simulink model "displayAlgorithm"  (R2015a)
settings: Solver=ode45  StartTime=0.0  StopTime=inf  RelTol=1e-3
InitFcn:
  | load busObjects
undefined symbols (not defined in the file or in its folder): gray
libraries: visiontextngfix x10, visionsinks x2, dspvision x1, sldrtlib x1
settings Model: Creator=sbiagion  LastModifiedBy=sbiagion
settings DebuggingCC: UnderspecifiedInitializationDetection=Classic  MergeDetectMultiDrivingBlocksExec=none  SolverPrmCheckMsg=warning

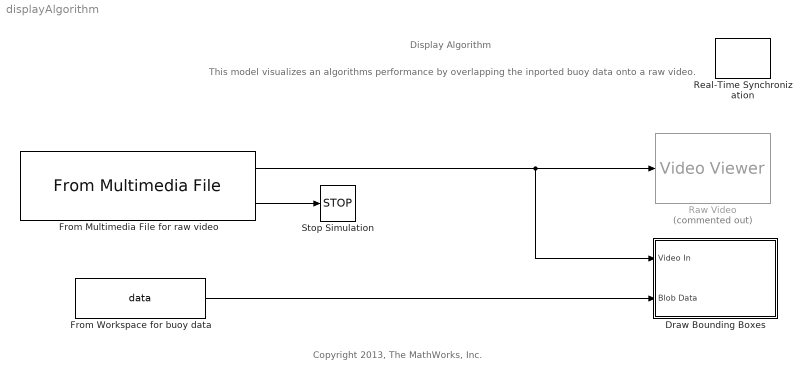
== system displayAlgorithm ==
  note: Copyright 2013, The MathWorks, Inc.
  note: This model visualizes an algorithms performance by overlapping the inported buoy data onto a raw video.
  note: Display Algorithm
  Draw Bounding Boxes : Subsystem
  From Multimedia File for raw video : dspvision/From Multimedia File  inputFilename=..\media\rawVideo_640x480.avi  loop=on  numPlays=1  outputStreams=Video only  videoDataType=uint8  audioDataType=int16  inheritSampleTime=on  userDefinedSampleTime=0.1  noAudioOutput=off  isIntensityVideo=off  fourcc=RGB  colorVideoFormat=One multidimensional signal  outputEOF=on  dataOrg=Column-major  audioFrameSize=1024  computeAudioFrameSize=off  outSamplingMode=Sample based
  From Workspace for buoy data : FromWorkspace  VariableName=data  OutDataTypeStr=Bus: dataBusObject
  "Raw Video " : visionsinks/Video Viewer  Commented=on  inputType=Obsolete7b  imagePorts=One multidimensional signal  useColorMap=off  colormapValue=gray(256)  specRange=off  minInputVal=0  maxInputVal=255  FigPos=[880 975 1008 708]  AxisZoom=on  trueSizedOnce=off  OpenAtMdlStart=on  DefaultConfigurationName=vipscopes.VideoViewerScopeCfg
  Real-Time Synchronization : sldrtlib/Real-Time Synchronization  SampleTime=0.1  MaxMissedTicks=1e9  ShowMissedTicks=off  YieldWhenWaiting=off
  Stop Simulation : Stop
  wires:
  From Workspace for buoy data/1 -> Draw Bounding Boxes/2(Blob Data)
  From Multimedia File for raw video/1 -> Draw Bounding Boxes/1(Video In), "Raw Video "/1
  From Multimedia File for raw video/2 -> Stop Simulation/1

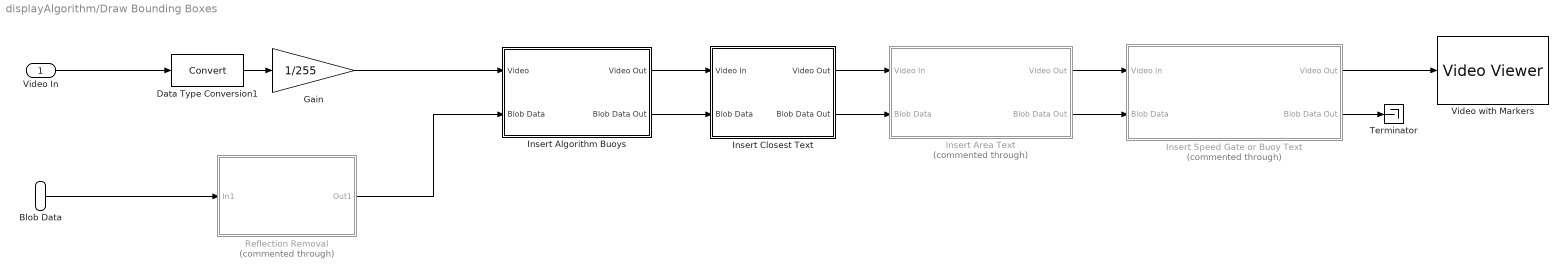
== system displayAlgorithm/Draw Bounding Boxes ==
  Video In : Inport
  Blob Data : Inport  Port=2
  Data Type Conversion1 : DataTypeConversion
  Gain : Gain  Gain=1/255
  Insert Algorithm Buoys : Subsystem
  Insert Area Text : Subsystem  Commented=through
  Insert Closest Text : Subsystem
  Insert Speed Gate or Buoy Text : Subsystem  Commented=through
  Reflection Removal : Subsystem  Commented=through
  Terminator : Terminator
  Video with Markers : visionsinks/Video Viewer  inputType=Obsolete7b  imagePorts=One multidimensional signal  useColorMap=off  colormapValue=gray(256)  specRange=off  minInputVal=0  maxInputVal=255  FigPos=[7 972 845 656]  AxisZoom=on  trueSizedOnce=off  OpenAtMdlStart=on  DefaultConfigurationName=vipscopes.VideoViewerScopeCfg
  wires:
  Data Type Conversion1/1 -> Gain/1
  Video In/1 -> Data Type Conversion1/1
  Insert Speed Gate or Buoy Text/1(Video Out) -> Video with Markers/1
  Insert Area Text/1(Video Out) -> Insert Speed Gate or Buoy Text/1(Video In)
  Insert Closest Text/1(Video Out) -> Insert Area Text/1(Video In)
  Reflection Removal/1(Out1) -> Insert Algorithm Buoys/2(Blob Data)
  Blob Data/1 -> Reflection Removal/1(In1)
  Gain/1 -> Insert Algorithm Buoys/1(Video)
  Insert Algorithm Buoys/1(Video Out) -> Insert Closest Text/1(Video In)
  Insert Algorithm Buoys/2(Blob Data Out) -> Insert Closest Text/2(Blob Data)
  Insert Closest Text/2(Blob Data Out) -> Insert Area Text/2(Blob Data)
  Insert Area Text/2(Blob Data Out) -> Insert Speed Gate or Buoy Text/2(Blob Data)
  Insert Speed Gate or Buoy Text/2(Blob Data Out) -> Terminator/1

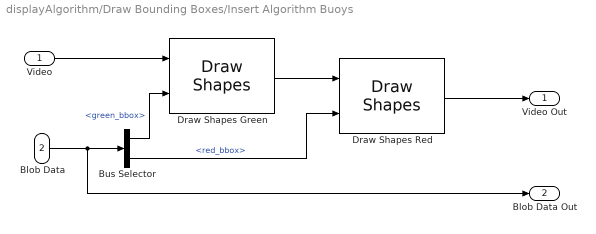
== system displayAlgorithm/Draw Bounding Boxes/Insert Algorithm Buoys ==
  Video : Inport
  Blob Data : Inport  Port=2
  Bus Selector : BusSelector  OutputSignals=green_bbox,red_bbox
  Draw Shapes Green : visiontextngfix/Draw Shapes  shape=Rectangles  fill=on  fillClrSource=Specify via dialog  display=User-specified value  intensity=200  color=[0 255 0]  opacity=0.6  viewport=Entire image  antialiasing=off  inType=Obsolete  imagePorts=One multidimensional signal  prodOutputMode=Binary point scaling  prodOutputWordLength=32  prodOutputFracLength=14  memoryMode=Specify word length  memoryWordLength=16  memoryFracLength=14  roundingMode=Floor  overflowMode=off
  Draw Shapes Red : visiontextngfix/Draw Shapes  shape=Rectangles  fill=on  fillClrSource=Specify via dialog  display=User-specified value  intensity=200  color=[255 0 0]  opacity=0.6  viewport=Entire image  antialiasing=off  inType=Obsolete  imagePorts=One multidimensional signal  prodOutputMode=Binary point scaling  prodOutputWordLength=32  prodOutputFracLength=14  memoryMode=Specify word length  memoryWordLength=16  memoryFracLength=14  roundingMode=Floor  overflowMode=off
  Video Out : Outport
  Blob Data Out : Outport  Port=2
  wires:
  Blob Data/1 -> Blob Data Out/1, Bus Selector/1
  Video/1 -> Draw Shapes Green/1
  Draw Shapes Green/1 -> Draw Shapes Red/1
  Draw Shapes Red/1 -> Video Out/1
  Bus Selector/1 -> Draw Shapes Green/2  "<green_bbox>"
  Bus Selector/2 -> Draw Shapes Red/2  "<red_bbox>"

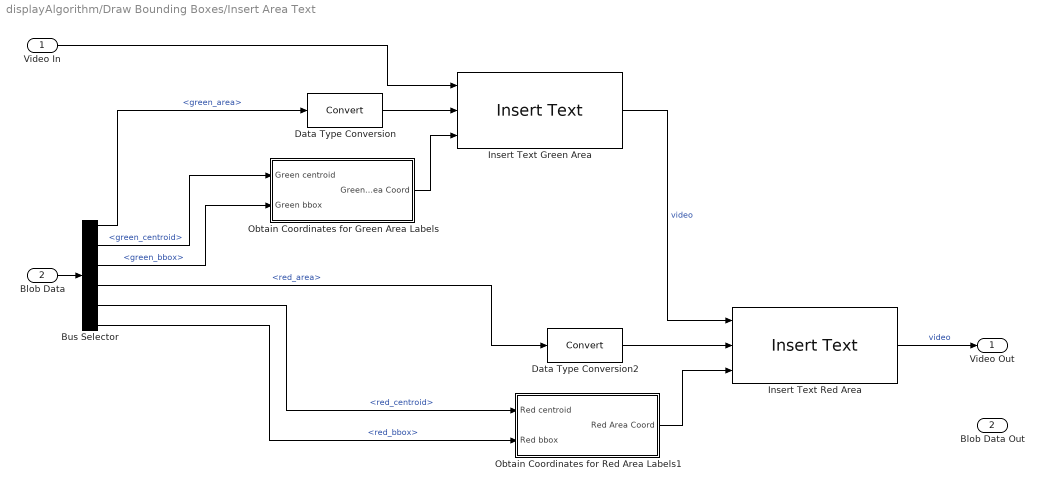
== system displayAlgorithm/Draw Bounding Boxes/Insert Area Text ==
  Video In : Inport
  Blob Data : Inport  Port=2
  Bus Selector : BusSelector  OutputSignals=green_area,green_centroid,green_bbox,red_area,red_centroid,red_bbox
  Data Type Conversion : DataTypeConversion
  Data Type Conversion2 : DataTypeConversion
  Insert Text Green Area : visiontextngfix/Insert Text  inputType=Obsolete  theText='Area: %d'  fontFace=LucidaSansRegular  dummyVar1=0  blockFontSize=12  antiAliased=on  getTextLocFrom=Input port  textLoc=[1 1]  getTextColorFrom=Specify via dialog  textColor=[0 255 0]  getTextIntensityFrom=Specify via dialog  textIntensity=0  getTextOpacityFrom=Specify via dialog  textOpacity=1.0  dummyVar2=0  dummyVar3=0  dummyVar4=0  imagePorts=One multidimensional signal  isInputTransposed=off
  Insert Text Red Area : visiontextngfix/Insert Text  inputType=Obsolete  theText='Area: %d'  fontFace=LucidaSansRegular  dummyVar1=0  blockFontSize=12  antiAliased=on  getTextLocFrom=Input port  textLoc=[1 1]  getTextColorFrom=Specify via dialog  textColor=[255 0 0]  getTextIntensityFrom=Specify via dialog  textIntensity=0  getTextOpacityFrom=Specify via dialog  textOpacity=1.0  dummyVar2=0  dummyVar3=0  dummyVar4=0  imagePorts=One multidimensional signal  isInputTransposed=off
  Obtain Coordinates for Green Area Labels : Subsystem
  Obtain Coordinates for Red Area Labels1 : Subsystem
  Video Out : Outport
  Blob Data Out : Outport  Port=2
  wires:
  Insert Text Red Area/1 -> Video Out/1  "video"
  Video In/1 -> Insert Text Green Area/1
  Bus Selector/4 -> Data Type Conversion2/1  "<red_area>"
  Bus Selector/1 -> Data Type Conversion/1  "<green_area>"
  Data Type Conversion/1 -> Insert Text Green Area/2
  Obtain Coordinates for Red Area Labels1/1(Red Area Coord) -> Insert Text Red Area/3
  Insert Text Green Area/1 -> Insert Text Red Area/1  "video"
  Data Type Conversion2/1 -> Insert Text Red Area/2
  Obtain Coordinates for Green Area Labels/1(Green Area Coord) -> Insert Text Green Area/3
  Blob Data/1 -> Bus Selector/1
  Bus Selector/2 -> Obtain Coordinates for Green Area Labels/1(Green centroid)  "<green_centroid>"
  Bus Selector/3 -> Obtain Coordinates for Green Area Labels/2(Green bbox)  "<green_bbox>"
  Bus Selector/5 -> Obtain Coordinates for Red Area Labels1/1(Red centroid)  "<red_centroid>"
  Bus Selector/6 -> Obtain Coordinates for Red Area Labels1/2(Red bbox)  "<red_bbox>"

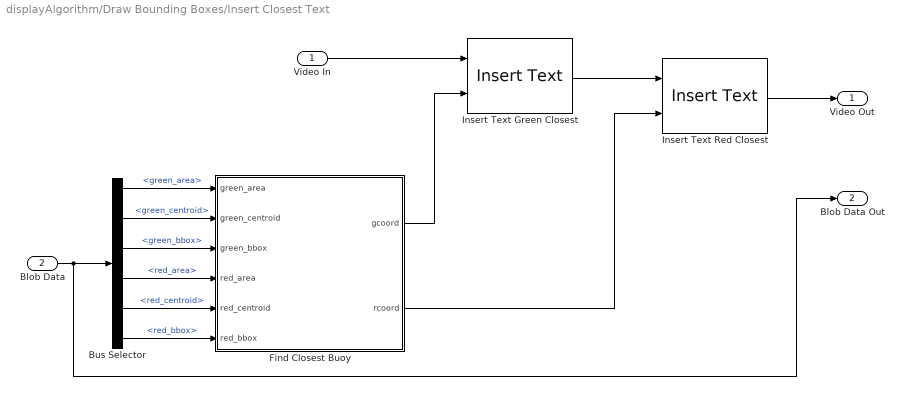
== system displayAlgorithm/Draw Bounding Boxes/Insert Closest Text ==
  Video In : Inport
  Blob Data : Inport  Port=2
  Bus Selector : BusSelector  OutputSignals=green_area,green_centroid,green_bbox,red_area,red_centroid,red_bbox
  Find Closest Buoy : MATLAB Function  TreatAsAtomicUnit=on
  Insert Text Green Closest : visiontextngfix/Insert Text  inputType=Obsolete  theText='Closest Green Buoy'  fontFace=LucidaSansRegular  dummyVar1=0  blockFontSize=12  antiAliased=on  getTextLocFrom=Input port  textLoc=[1 1]  getTextColorFrom=Specify via dialog  textColor=[0 255 0]  getTextIntensityFrom=Specify via dialog  textIntensity=0  getTextOpacityFrom=Specify via dialog  textOpacity=1.0  dummyVar2=0  dummyVar3=0  dummyVar4=0  imagePorts=One multidimensional signal  isInputTransposed=off
  Insert Text Red Closest : visiontextngfix/Insert Text  inputType=Obsolete  theText='Closest Red Buoy'  fontFace=LucidaSansRegular  dummyVar1=0  blockFontSize=12  antiAliased=on  getTextLocFrom=Input port  textLoc=[1 1]  getTextColorFrom=Specify via dialog  textColor=[255 0 0]  getTextIntensityFrom=Specify via dialog  textIntensity=0  getTextOpacityFrom=Specify via dialog  textOpacity=1.0  dummyVar2=0  dummyVar3=0  dummyVar4=0  imagePorts=One multidimensional signal  isInputTransposed=off
  Video Out : Outport
  Blob Data Out : Outport  Port=2
  wires:
  Insert Text Green Closest/1 -> Insert Text Red Closest/1
  Video In/1 -> Insert Text Green Closest/1
  Insert Text Red Closest/1 -> Video Out/1
  Find Closest Buoy/1(gcoord) -> Insert Text Green Closest/2
  Find Closest Buoy/2(rcoord) -> Insert Text Red Closest/2
  Blob Data/1 -> Blob Data Out/1, Bus Selector/1
  Bus Selector/3 -> Find Closest Buoy/3(green_bbox)  "<green_bbox>"
  Bus Selector/4 -> Find Closest Buoy/4(red_area)  "<red_area>"
  Bus Selector/2 -> Find Closest Buoy/2(green_centroid)  "<green_centroid>"
  Bus Selector/5 -> Find Closest Buoy/5(red_centroid)  "<red_centroid>"
  Bus Selector/1 -> Find Closest Buoy/1(green_area)  "<green_area>"
  Bus Selector/6 -> Find Closest Buoy/6(red_bbox)  "<red_bbox>"

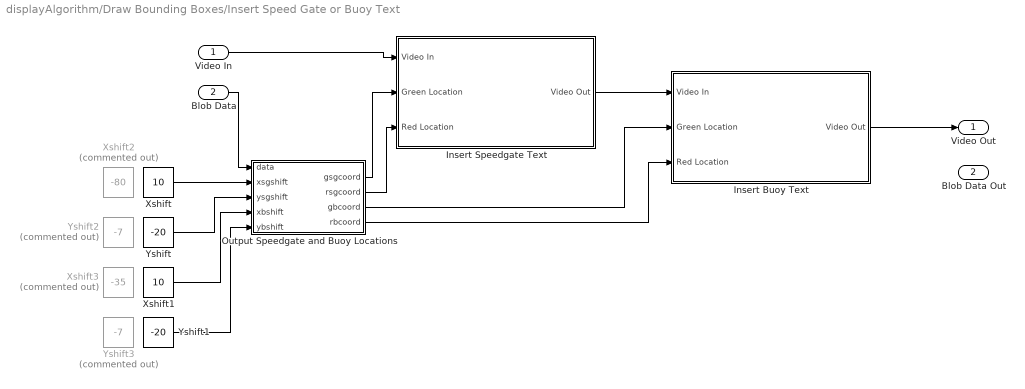
== system displayAlgorithm/Draw Bounding Boxes/Insert Speed Gate or Buoy Text ==
  Video In : Inport
  Blob Data : Inport  Port=2
  Insert Buoy Text : Subsystem
  Insert Speedgate Text : Subsystem
  Output Speedgate and Buoy Locations : MATLAB Function  TreatAsAtomicUnit=on
  Xshift : Constant  Value=10
  Xshift1 : Constant  Value=10
  Xshift2 : Constant  Commented=on  Value=-80
  Xshift3 : Constant  Commented=on  Value=-35
  Yshift : Constant  Value=-20
  Yshift1 : Constant  Value=-20
  Yshift2 : Constant  Commented=on  Value=-7
  Yshift3 : Constant  Commented=on  Value=-7
  Video Out : Outport
  Blob Data Out : Outport  Port=2
  wires:
  Video In/1 -> Insert Speedgate Text/1(Video In)
  Insert Speedgate Text/1(Video Out) -> Insert Buoy Text/1(Video In)
  Insert Buoy Text/1(Video Out) -> Video Out/1
  Blob Data/1 -> Output Speedgate and Buoy Locations/1(data)
  Output Speedgate and Buoy Locations/1(gsgcoord) -> Insert Speedgate Text/2(Green Location)
  Output Speedgate and Buoy Locations/2(rsgcoord) -> Insert Speedgate Text/3(Red Location)
  Output Speedgate and Buoy Locations/3(gbcoord) -> Insert Buoy Text/2(Green Location)
  Output Speedgate and Buoy Locations/4(rbcoord) -> Insert Buoy Text/3(Red Location)
  Xshift/1 -> Output Speedgate and Buoy Locations/2(xsgshift)
  Yshift/1 -> Output Speedgate and Buoy Locations/3(ysgshift)
  Xshift1/1 -> Output Speedgate and Buoy Locations/4(xbshift)
  Yshift1/1 -> Output Speedgate and Buoy Locations/5(ybshift)

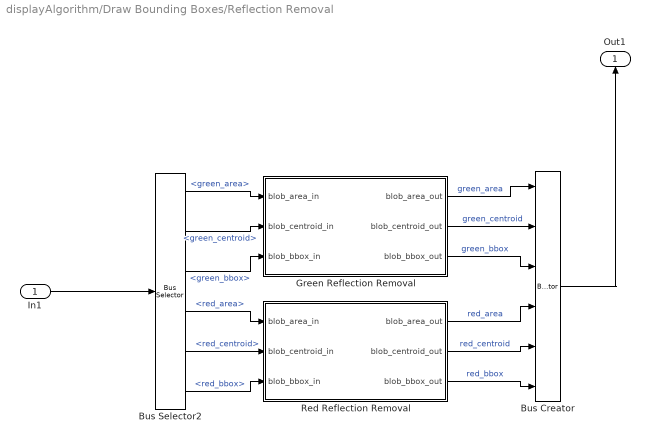
== system displayAlgorithm/Draw Bounding Boxes/Reflection Removal ==
  In1 : Inport
  Bus Creator : BusCreator  Inputs=6
  Bus Selector2 : BusSelector  OutputSignals=green_area,green_centroid,green_bbox,red_area,red_centroid,red_bbox
  Green Reflection Removal : MATLAB Function  TreatAsAtomicUnit=on
  Red Reflection Removal : MATLAB Function  TreatAsAtomicUnit=on
  Out1 : Outport
  wires:
  Red Reflection Removal/3(blob_bbox_out) -> Bus Creator/6  "red_bbox"
  Bus Selector2/1 -> Green Reflection Removal/1(blob_area_in)  "<green_area>"
  In1/1 -> Bus Selector2/1
  Bus Selector2/2 -> Green Reflection Removal/2(blob_centroid_in)  "<green_centroid>"
  Bus Selector2/4 -> Red Reflection Removal/1(blob_area_in)  "<red_area>"
  Bus Selector2/6 -> Red Reflection Removal/3(blob_bbox_in)  "<red_bbox>"
  Red Reflection Removal/2(blob_centroid_out) -> Bus Creator/5  "red_centroid"
  Green Reflection Removal/3(blob_bbox_out) -> Bus Creator/3  "green_bbox"
  Red Reflection Removal/1(blob_area_out) -> Bus Creator/4  "red_area"
  Bus Selector2/5 -> Red Reflection Removal/2(blob_centroid_in)  "<red_centroid>"
  Bus Creator/1 -> Out1/1
  Green Reflection Removal/1(blob_area_out) -> Bus Creator/1  "green_area"
  Bus Selector2/3 -> Green Reflection Removal/3(blob_bbox_in)  "<green_bbox>"
  Green Reflection Removal/2(blob_centroid_out) -> Bus Creator/2  "green_centroid"

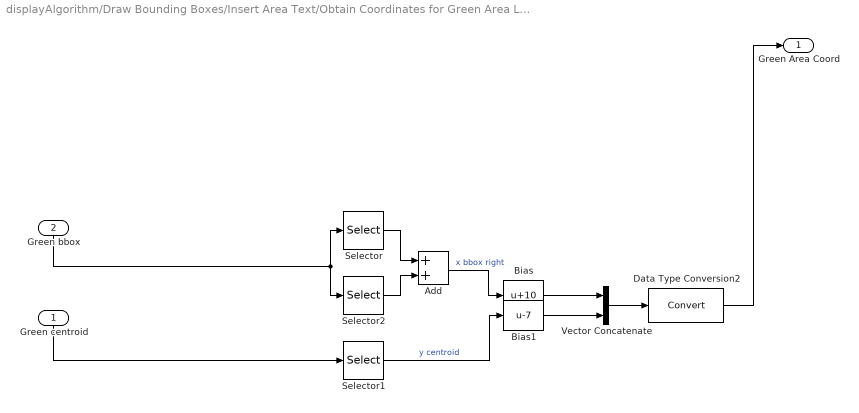
== system displayAlgorithm/Draw Bounding Boxes/Insert Area Text/Obtain Coordinates for Green Area Labels ==
  Green centroid : Inport
  Green bbox : Inport  Port=2
  Add : Sum
  Bias : Bias  Bias=10
  Bias1 : Bias  Bias=-7
  Data Type Conversion2 : DataTypeConversion
  Selector : Selector  NumberOfDimensions=2  InputPortWidth=3  IndexOptions=Select all,Index vector (dialog)  Indices=[1 3],1  OutputSizes=1,1
  Selector1 : Selector  NumberOfDimensions=2  InputPortWidth=3  IndexOptions=Select all,Index vector (dialog)  Indices=[1 3],2  OutputSizes=1,1
  Selector2 : Selector  NumberOfDimensions=2  InputPortWidth=3  IndexOptions=Select all,Index vector (dialog)  Indices=[1 3],3  OutputSizes=1,1
  Vector Concatenate : Concatenate  Mode=Multidimensional array  ConcatenateDimension=2
  Green Area Coord : Outport
  wires:
  Selector1/1 -> Bias1/1  "y centroid"
  Selector2/1 -> Add/2
  Vector Concatenate/1 -> Data Type Conversion2/1
  Add/1 -> Bias/1  "x bbox right"
  Selector/1 -> Add/1
  Bias/1 -> Vector Concatenate/1
  Data Type Conversion2/1 -> Green Area Coord/1
  Bias1/1 -> Vector Concatenate/2
  Green bbox/1 -> Selector2/1, Selector/1
  Green centroid/1 -> Selector1/1

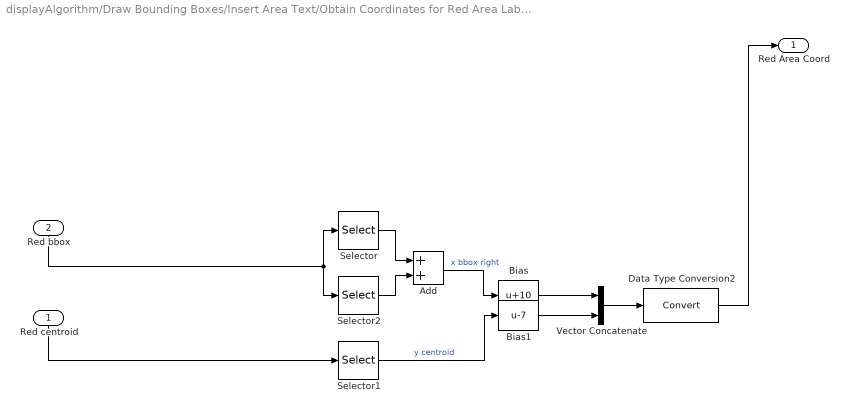
== system displayAlgorithm/Draw Bounding Boxes/Insert Area Text/Obtain Coordinates for Red Area Labels1 ==
  Red centroid : Inport
  Red bbox : Inport  Port=2
  Add : Sum
  Bias : Bias  Bias=10
  Bias1 : Bias  Bias=-7
  Data Type Conversion2 : DataTypeConversion
  Selector : Selector  NumberOfDimensions=2  InputPortWidth=3  IndexOptions=Select all,Index vector (dialog)  Indices=[1 3],1  OutputSizes=1,1
  Selector1 : Selector  NumberOfDimensions=2  InputPortWidth=3  IndexOptions=Select all,Index vector (dialog)  Indices=[1 3],2  OutputSizes=1,1
  Selector2 : Selector  NumberOfDimensions=2  InputPortWidth=3  IndexOptions=Select all,Index vector (dialog)  Indices=[1 3],3  OutputSizes=1,1
  Vector Concatenate : Concatenate  Mode=Multidimensional array  ConcatenateDimension=2
  Red Area Coord : Outport
  wires:
  Red centroid/1 -> Selector1/1
  Red bbox/1 -> Selector/1, Selector2/1
  Bias1/1 -> Vector Concatenate/2
  Data Type Conversion2/1 -> Red Area Coord/1
  Bias/1 -> Vector Concatenate/1
  Selector/1 -> Add/1
  Add/1 -> Bias/1  "x bbox right"
  Vector Concatenate/1 -> Data Type Conversion2/1
  Selector2/1 -> Add/2
  Selector1/1 -> Bias1/1  "y centroid"

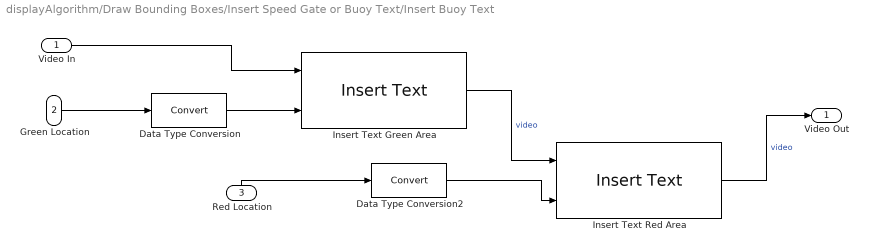
== system displayAlgorithm/Draw Bounding Boxes/Insert Speed Gate or Buoy Text/Insert Buoy Text ==
  Video In : Inport
  Green Location : Inport  Port=2
  Red Location : Inport  Port=3
  Data Type Conversion : DataTypeConversion
  Data Type Conversion2 : DataTypeConversion
  Insert Text Green Area : visiontextngfix/Insert Text  inputType=Obsolete  theText='Buoy'  fontFace=LucidaSansRegular  dummyVar1=0  blockFontSize=12  antiAliased=on  getTextLocFrom=Input port  textLoc=[1 1]  getTextColorFrom=Specify via dialog  textColor=[0 255 0]  getTextIntensityFrom=Specify via dialog  textIntensity=0  getTextOpacityFrom=Specify via dialog  textOpacity=1.0  dummyVar2=0  dummyVar3=0  dummyVar4=0  imagePorts=One multidimensional signal  isInputTransposed=off
  Insert Text Red Area : visiontextngfix/Insert Text  inputType=Obsolete  theText='Buoy'  fontFace=LucidaSansRegular  dummyVar1=0  blockFontSize=12  antiAliased=on  getTextLocFrom=Input port  textLoc=[1 1]  getTextColorFrom=Specify via dialog  textColor=[255 0 0]  getTextIntensityFrom=Specify via dialog  textIntensity=0  getTextOpacityFrom=Specify via dialog  textOpacity=1.0  dummyVar2=0  dummyVar3=0  dummyVar4=0  imagePorts=One multidimensional signal  isInputTransposed=off
  Video Out : Outport
  wires:
  Insert Text Red Area/1 -> Video Out/1  "video"
  Video In/1 -> Insert Text Green Area/1
  Red Location/1 -> Data Type Conversion2/1
  Green Location/1 -> Data Type Conversion/1
  Data Type Conversion/1 -> Insert Text Green Area/2
  Insert Text Green Area/1 -> Insert Text Red Area/1  "video"
  Data Type Conversion2/1 -> Insert Text Red Area/2

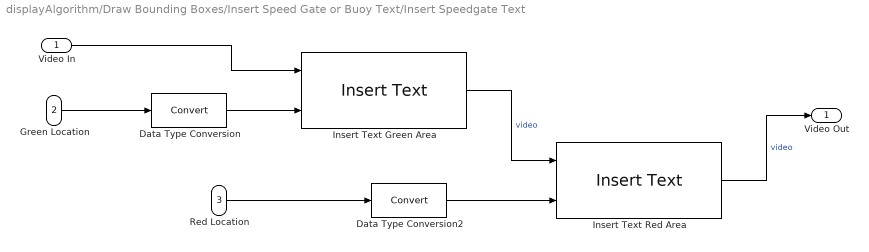
== system displayAlgorithm/Draw Bounding Boxes/Insert Speed Gate or Buoy Text/Insert Speedgate Text ==
  Video In : Inport
  Green Location : Inport  Port=2
  Red Location : Inport  Port=3
  Data Type Conversion : DataTypeConversion
  Data Type Conversion2 : DataTypeConversion
  Insert Text Green Area : visiontextngfix/Insert Text  inputType=Obsolete  theText='Speed Gate'  fontFace=LucidaSansRegular  dummyVar1=0  blockFontSize=12  antiAliased=on  getTextLocFrom=Input port  textLoc=[1 1]  getTextColorFrom=Specify via dialog  textColor=[0 255 0]  getTextIntensityFrom=Specify via dialog  textIntensity=0  getTextOpacityFrom=Specify via dialog  textOpacity=1.0  dummyVar2=0  dummyVar3=0  dummyVar4=0  imagePorts=One multidimensional signal  isInputTransposed=off
  Insert Text Red Area : visiontextngfix/Insert Text  inputType=Obsolete  theText='Speed Gate'  fontFace=LucidaSansRegular  dummyVar1=0  blockFontSize=12  antiAliased=on  getTextLocFrom=Input port  textLoc=[1 1]  getTextColorFrom=Specify via dialog  textColor=[255 0 0]  getTextIntensityFrom=Specify via dialog  textIntensity=0  getTextOpacityFrom=Specify via dialog  textOpacity=1.0  dummyVar2=0  dummyVar3=0  dummyVar4=0  imagePorts=One multidimensional signal  isInputTransposed=off
  Video Out : Outport
  wires:
  Data Type Conversion2/1 -> Insert Text Red Area/2
  Insert Text Green Area/1 -> Insert Text Red Area/1  "video"
  Data Type Conversion/1 -> Insert Text Green Area/2
  Green Location/1 -> Data Type Conversion/1
  Red Location/1 -> Data Type Conversion2/1
  Video In/1 -> Insert Text Green Area/1
  Insert Text Red Area/1 -> Video Out/1  "video"

== matlab function displayAlgorithm/Draw Bounding Boxes/Reflection Removal/Green Reflection Removal ==
  data: blob_area_in input; blob_centroid_in input; blob_bbox_in input; blob_area_out output; blob_centroid_out output; blob_bbox_out output
function [blob_area_out, blob_centroid_out, blob_bbox_out] = fcn(blob_area_in,blob_centroid_in, blob_bbox_in)
%#codegen
%% buoy reflection removal 

% extract valid blob data
blobidx = find(blob_centroid_in(:,1)~=-1); % locations in original vector where blob data is
nblobs = length(blobidx);

blob_area = blob_area_in(blobidx,:);
blob_centroid = double(blob_centroid_in(blobidx,:)); 
blob_bbox = blob_bbox_in(blobidx,:);

% only perform blob reflection removal if there are more than 1 blobs
if nblobs >=2
    tolXC = 80;
    connectivity = zeros(1,2);
    diffXC = zeros(1,2);

    % create difference and connectivity matrix
    % diffXC = absolute difference between X coordinates of centroids
    % connectivity matrix provides all of the comparisons that can be performed
    if nblobs == 2
        diffXC = abs(blob_centroid(1,1)-blob_centroid(2,1));
        connectivity = [1 2];  
    elseif nblobs == 3
        diffXC = abs([blob_centroid(1,1)-blob_centroid(2,1);
                        blob_centroid(1,1)-blob_centroid(3,1);
                        blob_centroid(2,1)-blob_centroid(3,1)]);
        connectivity = [1 2; 1 3; 2 3];
    elseif nblobs == 4
        diffXC = abs([blob_centroid(1,1)-blob_centroid(2,1);
                        blob_centroid(1,1)-blob_centroid(3,1);
                        blob_centroid(1,1)-blob_centroid(4,1);
                        blob_centroid(2,1)-blob_centroid(3,1);
                        blob_centroid(2,1)-blob_centroid(4,1);
                        blob_centroid(3,1)-blob_centroid(4,1)]);
        connectivity = [1 2; 1 3; 1 4; 2 3; 2 4; 3 4];
    end

    % loop through connectivity matrix to find reflection blobs and remove
    boolXC = diffXC<tolXC;
    for idx = 1:size(connectivity,1);
        if boolXC(idx)
           % remove lower blob corresponding to connectivity(idx,:)
           % find lower blob
           refidx = connectivity(idx,:); % i.e. [1 2] buoys which are possibly reflections

           [~,maxidx] = max(blob_centroid(refidx,2)); % i.e. [2] % buoy which is lowest aka reflection
           [~,minidx] = min(blob_centroid(refidx,2)); 
           
           if blob_area(refidx(maxidx))<blob_area(refidx(minidx)) % if lowest blob's area is smaller than upper blob, remove
               % erase blob data corresponding to reflections
               blob_area(blobidx(refidx(maxidx)),:) = -1;
               blob_centroid(blobidx(refidx(maxidx)),:) = -1;
               blob_bbox(blobidx(refidx(maxidx)),:) = -1;
           end
           % blobidx(refidx) = [2 3];
           % blobidx(refidx(maxidx) = 2;
        end
    end  
end % end of blob removal

% color specific 
% output red data
blob_area_out = -ones(4,1);
blob_centroid_out = -ones(4,2);
blob_bbox_out = -ones(4,4);

blob_area_out(1:nblobs) = blob_area;
blob_centroid_out(1:nblobs,:) = blob_centroid;
blob_bbox_out(1:nblobs,:) = blob_bbox;

== matlab function displayAlgorithm/Draw Bounding Boxes/Reflection Removal/Red Reflection Removal ==
  data: blob_area_in input; blob_centroid_in input; blob_bbox_in input; blob_area_out output; blob_centroid_out output; blob_bbox_out output
function [blob_area_out, blob_centroid_out, blob_bbox_out] = fcn(blob_area_in,blob_centroid_in, blob_bbox_in)
%#codegen
%% buoy reflection removal 

% extract valid blob data
blobidx = find(blob_centroid_in(:,1)~=-1); % locations in original vector where blob data is
nblobs = length(blobidx);

blob_area = blob_area_in(blobidx,:);
blob_centroid = double(blob_centroid_in(blobidx,:)); 
blob_bbox = blob_bbox_in(blobidx,:);

% only perform blob reflection removal if there are more than 1 blobs
if nblobs >=2
    tolXC = 20;
    connectivity = zeros(1,2);
    diffXC = zeros(1,2);

    % create difference and connectivity matrix
    % diffXC = absolute difference between X coordinates of centroids
    % connectivity matrix provides all of the comparisons that can be performed
    if nblobs == 2
        diffXC = abs(blob_centroid(1,1)-blob_centroid(2,1));
        connectivity = [1 2];  
    elseif nblobs == 3
        diffXC = abs([blob_centroid(1,1)-blob_centroid(2,1);
                        blob_centroid(1,1)-blob_centroid(3,1);
                        blob_centroid(2,1)-blob_centroid(3,1)]);
        connectivity = [1 2; 1 3; 2 3];
    elseif nblobs == 4
        diffXC = abs([blob_centroid(1,1)-blob_centroid(2,1);
                        blob_centroid(1,1)-blob_centroid(3,1);
                        blob_centroid(1,1)-blob_centroid(4,1);
                        blob_centroid(2,1)-blob_centroid(3,1);
                        blob_centroid(2,1)-blob_centroid(4,1);
                        blob_centroid(3,1)-blob_centroid(4,1)]);
        connectivity = [1 2; 1 3; 1 4; 2 3; 2 4; 3 4];
    end

    % loop through connectivity matrix to find reflection blobs and remove
    boolXC = diffXC<tolXC;
    for idx = 1:size(connectivity,1);
        if boolXC(idx)
           % remove lower blob corresponding to connectivity(idx,:)
           % find lower blob
           refidx = connectivity(idx,:); % i.e. [1 2] buoys which are possibly reflections

           [~,maxidx] = max(blob_centroid(refidx,2)); % i.e. [2] % buoy which is lowest aka reflection
           [~,minidx] = min(blob_centroid(refidx,2)); 
           
           if blob_area(refidx(maxidx))<blob_area(refidx(minidx)) % if lowest blob's area is smaller than upper blob, remove
               % erase blob data corresponding to reflections
               blob_area(blobidx(refidx(maxidx)),:) = -1;
               blob_centroid(blobidx(refidx(maxidx)),:) = -1;
               blob_bbox(blobidx(refidx(maxidx)),:) = -1;
           end
           % blobidx(refidx) = [2 3];
           % blobidx(refidx(maxidx) = 2;
        end
    end  
end % end of blob removal

% color specific 
% output red data
blob_area_out = -ones(4,1);
blob_centroid_out = -ones(4,2);
blob_bbox_out = -ones(4,4);

blob_area_out(1:nblobs) = blob_area;
blob_centroid_out(1:nblobs,:) = blob_centroid;
blob_bbox_out(1:nblobs,:) = blob_bbox;

== matlab function displayAlgorithm/Draw Bounding Boxes/Insert Closest Text/Find Closest Buoy ==
  data: green_area input; green_centroid input; gcoord output; green_bbox input; red_area input; red_centroid input; red_bbox input; rcoord output
function [gcoord, rcoord] = fcn(green_area,green_centroid,green_bbox,red_area,red_centroid,red_bbox)
%#codegen

% identify and remove buoys from the second track


trackID = 1; % 1 == left track, 2 == right track
if trackID==1
    % if boat is on left track remove red buoys to the right of the green
    % speed gates
    % determine which blob is a speed gate
    gh = green_bbox(:,4);
    gw = green_bbox(:,3);
    % gsgidx = Green Speed Gate Idx, points to the buoys which are green
    % speed gates
    gsgidx = find(green_area>500 & gh-gw>30);
    if ~isempty(gsgidx)
        gr = green_bbox(gsgidx(1),1)+green_bbox(gsgidx(1),3);
        % find red buoys that are on the second track and remove them
        rl = red_bbox(:,1);
        rstidx = find(rl>gr); 
        red_area(rstidx) = -1;
        red_centroid(rstidx,:) = -1;
        red_bbox(rstidx,:) = -1;
    end
end

[~, green_closestBuoyIdx] = max(green_bbox(:,2)+green_bbox(:,4));
gcoord = int16([green_centroid(green_closestBuoyIdx,1)-20 green_bbox(green_closestBuoyIdx,2)-15]);

[~, red_closestBuoyIdx] = max(red_bbox(:,2)+red_bbox(:,4));
rcoord = int16([red_centroid(red_closestBuoyIdx,1)-20 red_bbox(red_closestBuoyIdx,2)-15]);

== matlab function displayAlgorithm/Draw Bounding Boxes/Insert Speed Gate or Buoy Text/Output Speedgate and Buoy Locations ==
  data: data input Bus: dataBusObject; gsgcoord output size=[4 2]; rsgcoord output size=[4 2]; xsgshift input; ysgshift input; gbcoord output size=[4 2]; rbcoord output size=[4 2]; xbshift input; ybshift input
function [gsgcoord,rsgcoord,gbcoord,rbcoord]= fcn(data,xsgshift,ysgshift,xbshift,ybshift)
%#codegen
    % define thresholds
    athreshold = 500;
    hwthreshold = 25;

    % determine which green blob is a speed gate
    gh = data.green_bbox(:,4);
    gw = data.green_bbox(:,3);
    % gsgidx = Green Speed Gate Idx, points to the buoys which are green
    % speed gates
    
    gsgidx = find(data.green_area>athreshold & gh-gw>hwthreshold);
    gsgcoord = [data.green_bbox(gsgidx,1)+gw(gsgidx)+xsgshift data.green_centroid(gsgidx,2)+ysgshift];
    gbidx = find(gh-gw<hwthreshold);
    gbcoord = [data.green_bbox(gbidx,1)+gw(gbidx)+xbshift data.green_centroid(gbidx,2)+ybshift];
    
    % determine which red blob is a speed gate
    rh = data.red_bbox(:,4);
    rw = data.red_bbox(:,3);
    % gsgidx = red Speed Gate Idx, points to the buoys which are red
    % speed gates
    rsgidx = find(data.red_area>athreshold & rh-rw>hwthreshold);
    rsgcoord = [data.red_bbox(rsgidx,1)+rw(rsgidx)+xsgshift data.red_centroid(rsgidx,2)+ysgshift];
    rbidx = find(rh-rw<hwthreshold);
    rbcoord = [data.red_bbox(rbidx,1)++rw(rbidx)+xbshift data.red_centroid(rbidx,2)+ybshift];
